simulink model "mixed"  (Simulink 4.00)
settings: Solver=ode5  SolverMode=SingleTasking  StartTime=0.0  StopTime=10  FixedStep=.1  MaxStep=.1  RelTol=1e-3  AbsTol=1e-6
settings Model: CovMetricSettings=d  Creator=ciolfi  LastModifiedBy=ciolfi  ExternalInput=[]  InitialState=[]  LimitDataPoints=off  IntegerOverflowMsg=none  ExtModeTrigMode=oneshot  ExtModeArmWhenConnect=off  ExtModeAutoUpdateStatusClock=off

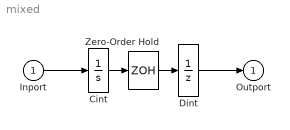
== system mixed ==
  Inport : Inport  Port=1  LatchInput=off
  Cint : Integrator  ExternalReset=none  InitialConditionSource=internal  InitialCondition=1  LimitOutput=off  UpperSaturationLimit=inf  LowerSaturationLimit=-inf  ShowSaturationPort=off  ShowStatePort=off  AbsoluteTolerance=auto
  Dint : UnitDelay  X0=1  SampleTime=1
      settings: RTWStateStorageClass=Auto
  Zero-Order Hold : ZeroOrderHold  SampleTime=1
  Outport : Outport  Port=1  InitialOutput=0
  wires:
  Dint/1 -> Outport/1
  Inport/1 -> Cint/1
  Cint/1 -> Zero-Order Hold/1
  Zero-Order Hold/1 -> Dint/1
